simulink model "Week3_Problem2"  (R2020a)
settings: Solver=VariableStepAuto  StartTime=0.0  StopTime=10.0  RelTol=1e-3
settings Model: Creator=tnradm  LastModifiedBy=tnradm

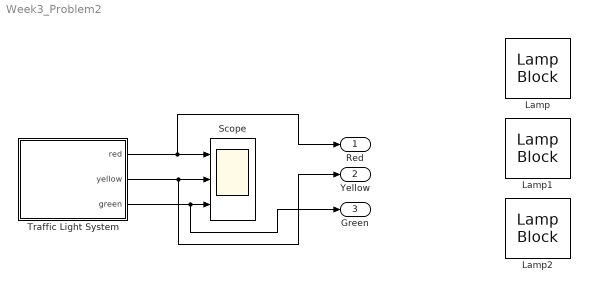
== system Week3_Problem2 ==
  Lamp : LampBlock
  Lamp1 : LampBlock
  Lamp2 : LampBlock
  Scope : Scope  NumInputPorts=3
  Traffic Light System : Stateflow chart  TreatAsAtomicUnit=on
  Red : Outport
  Yellow : Outport  Port=2
  Green : Outport  Port=3
  wires:
  Traffic Light System/1(red) -> Red/1, Scope/1
  Traffic Light System/2(yellow) -> Yellow/1, Scope/2
  Traffic Light System/3(green) -> Green/1, Scope/3

== stateflow chart Week3_Problem2/Traffic Light System ==
  state Prepare
    entry:red=0;
    green=0;
    yellow=1;
  state Go
    entry:yellow=0;
    red=0;
    green=1;
    flag=1;
  state Stop
    entry:yellow=0;
    green=0;
    red=1;
    flag=0;
  (default) -> Stop
  Prepare -> Go [order 1] : [flag==0]
  Stop -> Prepare : [after(2,sec)]
  Prepare -> Stop [order 2] : [flag==1]
  Go -> Prepare : [after(2,sec)]
  data: red output; yellow output; green output; flag local
